simulink model "runGantrySimulink"  (R2025b)
settings: Solver=FixedStepAuto  StartTime=0.0  StopTime=inf  FixedStep=0.05  RelTol=1e-3  EnableMultiTasking=on
libraries: raspberrypiNetworklib x4, raspberrypiBasiclib x4, etargetslib x2
settings Model: ExtModeTrigDuration=2  Creator=ioannisgeorgilas  LastModifiedBy=james
settings SolverCC: PositivePriorityOrder=on
settings OptimizationCC: EnhancedBackFolding=on  PassReuseOutputArgsAs=Individual arguments  ZeroExternalMemoryAtStartup=off  ZeroInternalMemoryAtStartup=off  MaxStackSize=200000  OptimizeBlockOrder=speed  DifferentSizesBufferReuse=on  OptimizationCustomize=off  EfficientTunableParamExpr=on
settings DebuggingCC: ParameterTunabilityLossMsg=error
settings HardwareCC: ProdBitPerPointer=32.0  ProdBitPerSizeT=32.0  ProdBitPerPtrDiffT=32.0  ProdLargestAtomicInteger=Long  ProdLargestAtomicFloat=Double  ProdWordSize=32.0  ProdLongLongMode=on  ProdHWDeviceType=ARM Compatible->ARM Cortex-A (32-bit)
settings RTWCC: SystemTargetFile=ert.tlc  HardwareBoard=Raspberry Pi  TLCOptions="-aInlineSetEventsForThisBaseRateFcn=TLC_FALSE -aSuppressMultiTaskScheduler=TLC_FALSE  -aRateBasedStepFcn=0"  TemplateMakefile=ert_default_tmf  Toolchain=GNU GCC Embedded Linux  BuildConfiguration=Faster Runs  Description=Embedded Coder
settings CodeAppCC: ForceParamTrailComments=on  IgnoreCustomStorageClasses=off  OperatorAnnotations=on  SimulinkDataObjDesc=on  SFDataObjDesc=on  InsertBlockDesc=on
settings ERTTargetCC: ExtModeTransport=2.0  ExtModeStaticAlloc=on  ExtModeMexFile=ext_xcp  ExtModeIntrfLevel=Level2 - Open  InlinedParameterPlacement=Hierarchical  CodeReplacementLibrary=ARM Cortex-A CMSIS  SupportContinuousTime=on  SupportVariableSizeSignals=on

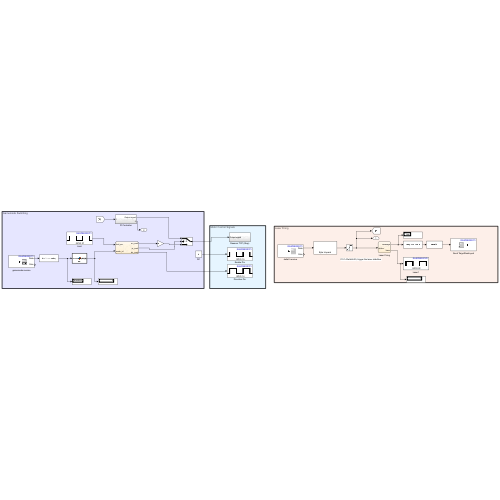
[thumbnail: Simulink's stored preview of the top-level diagram]
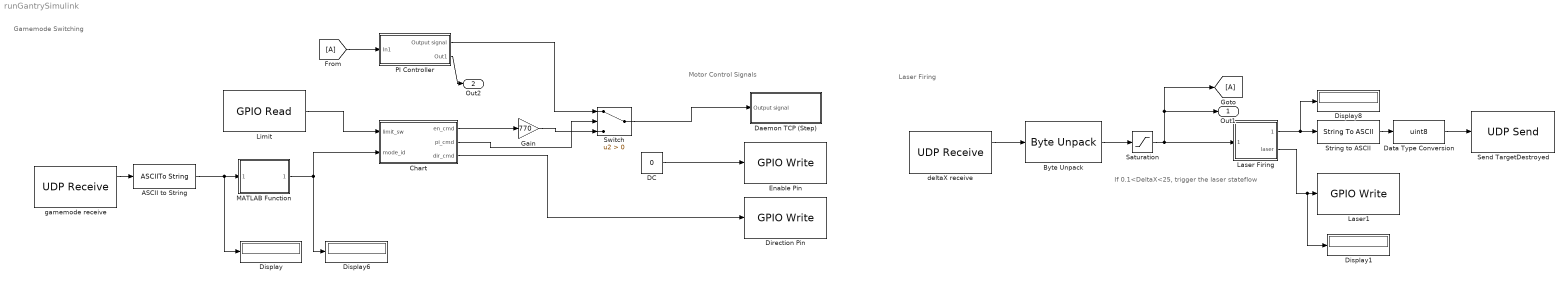
== system runGantrySimulink ==
  note: If 0.1<DeltaX<25, trigger the laser stateflow
  note: Motor Control Signals
  note: Laser Firing
  note: Gamemode Switching
  ASCII to String : ASCIIToString
  Byte Unpack : etargetslib/Byte Unpack  dimensions={[1]}  datatypes={'int32'}  byteAlign=1
      settings: LibrarySourceBlock=embeddedtargetslib/Host Communication/Byte Unpack
  Chart : Stateflow chart  TreatAsAtomicUnit=on
  DC : Constant  Value=0
  Daemon TCP (Step) : Subsystem
  Data Type Conversion : DataTypeConversion  OutDataTypeStr=uint8  SaturateOnIntegerOverflow=off  RndMeth=Floor
  Direction Pin : raspberrypiBasiclib/GPIO Write  BoardProperty=Pi Zero 2 W  gpio=14  blockPlatform=Raspberry Pi  PinNumber=17  board=[]  direction=[]
  Display{,1,6,8} (4 alike) : Display
  Enable Pin : raspberrypiBasiclib/GPIO Write  BoardProperty=Pi Zero 2 W  gpio=15  blockPlatform=Raspberry Pi  PinNumber=17  board=[]  direction=[]
  From : From
  Gain : Gain  Gain=770
  Goto : Goto
  Laser Firing : Stateflow chart  TreatAsAtomicUnit=on
  Laser1 : raspberrypiBasiclib/GPIO Write  BoardProperty=Pi Zero 2 W  gpio=22  blockPlatform=Raspberry Pi  PinNumber=17  board=[]  direction=[]
  Limit : raspberrypiBasiclib/GPIO Read  BoardProperty=Pi Zero 2 W  gpio=27  SampleTime=0.05  blockPlatform=Raspberry Pi  PinNumber=4  board=[]  direction=[]  internalResistor=[]
  MATLAB Function : MATLAB Function  TreatAsAtomicUnit=on
  PI Controller : Subsystem
  Saturation : Saturate  UpperLimit=500  LowerLimit=-500
  Send TargetDestroyed : raspberrypiNetworklib/UDP Send  remoteURL='172.26.236.65'  remotePort=55004  localURL='0.0.0.0'  localPortSource=Automatically determine  localPort=-1  sampletime=-1  blockPlatform=Raspberry Pi  separateLengthPort=0
  String to ASCII : StringToASCII
  Switch : Switch  Criteria=u2 > Threshold  SaturateOnIntegerOverflow=off  InputSameDT=off
  deltaX receive : raspberrypiNetworklib/UDP Receive  localURL='0.0.0.0'  localPort=55010  remoteURL='0.0.0.0'  remotePort=-1  recvBufferSize=8192  signalDatatype=uint8  dims=4  isVarSize=off  showBlockingTime=off  blockingTime=0  sampletime=0.05  blockPlatform=Raspberry Pi
  gamemode receive : raspberrypiNetworklib/UDP Receive  localURL='0.0.0.0'  localPort=50001  remoteURL='0.0.0.0'  remotePort=-1  recvBufferSize=8192  signalDatatype=uint8  dims=14  isVarSize=off  showBlockingTime=off  blockingTime=0  sampletime=0.05  blockPlatform=Raspberry Pi
  Out1 : Outport
  Out2 : Outport  Port=2
  wires:
  Chart/3(dir_cmd) -> Direction Pin/1
  ASCII to String/1 -> MATLAB Function/1(command_string), Display/1
  Limit/1 -> Chart/1(limit_sw)
  DC/1 -> Enable Pin/1
  MATLAB Function/1(mode_id) -> Chart/2(mode_id), Display6/1
  gamemode receive/1 -> ASCII to String/1
  deltaX receive/1 -> Byte Unpack/1
  Byte Unpack/1 -> Saturation/1
  Saturation/1 -> Laser Firing/1(deltax), Goto/1, Out1/1
  Data Type Conversion/1 -> Send TargetDestroyed/1
  Laser Firing/1(message) -> Display8/1, String to ASCII/1
  String to ASCII/1 -> Data Type Conversion/1
  Chart/2(pi_cmd) -> Switch/2
  PI Controller/1(Output signal) -> Switch/1
  PI Controller/2(Out1) -> Out2/1
  Switch/1 -> Daemon TCP (Step)/1(Output signal)
  Chart/1(en_cmd) -> Gain/1
  Gain/1 -> Switch/3
  From/1 -> PI Controller/1(In1)
  Laser Firing/2(laser) -> Display1/1, Laser1/1

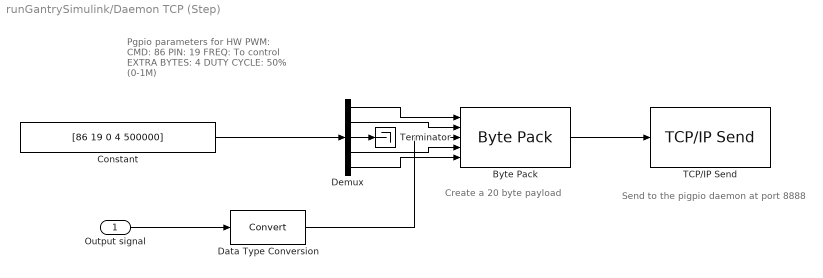
== system runGantrySimulink/Daemon TCP (Step) ==
  note: Pgpio parameters for HW PWM:
      | CMD: 86
      | PIN: 19
      | FREQ: To control
      | EXTRA BYTES: 4
      | DUTY CYCLE: 50% (0-1M)
  note: Create a 20 byte payload
  note: Send to the pigpio daemon at port 8888
  Output signal : Inport
  Byte Pack : etargetslib/Byte Pack  datatypes={'uint32','uint32','uint32','uint32','uint32'}  byteAlign=1
  Constant : Constant  Value=[86 19 0 4 500000]  OutDataTypeStr=Inherit: Inherit via back propagation
  Data Type Conversion : DataTypeConversion  SaturateOnIntegerOverflow=off  RndMeth=Floor
  Demux : Demux  Outputs=5
  TCP/IP Send : raspberrypiNetworklib/TCP//IP Send  Mode_=Client  LocalServerPort_=25000  RemoteAddr_=127.0.0.1  RemoteServerPort_=8888  SimulateUsing=Code generation  ClientPortBindingSelection_=off  ClientPortToBind_=35000  BlockingMode_=off  BlockTimeout_=0.1  BlockPlatform=RASPBERRYPI
  Terminator : Terminator
  wires:
  Byte Pack/1 -> TCP/IP Send/1
  Demux/1 -> Byte Pack/1
  Demux/2 -> Byte Pack/2
  Demux/3 -> Terminator/1
  Demux/4 -> Byte Pack/4
  Demux/5 -> Byte Pack/5
  Data Type Conversion/1 -> Byte Pack/3
  Constant/1 -> Demux/1
  Output signal/1 -> Data Type Conversion/1

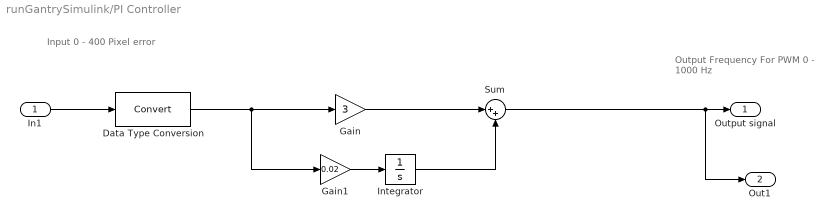
== system runGantrySimulink/PI Controller ==
  note: Output Frequency For PWM
      | 0 - 1000 Hz
  note: Input 0 - 400 Pixel error
  In1 : Inport
  Data Type Conversion : DataTypeConversion  SaturateOnIntegerOverflow=off  RndMeth=Floor
  Gain : Gain  Gain=3
  Gain1 : Gain  Gain=0.02
  Integrator : Integrator
  Sum : Sum  Inputs=|++
  Output signal : Outport
  Out1 : Outport  Port=2
  wires:
  Data Type Conversion/1 -> Gain1/1, Gain/1
  Gain1/1 -> Integrator/1
  Gain/1 -> Sum/1
  Integrator/1 -> Sum/2
  Sum/1 -> Out1/1, Output signal/1
  In1/1 -> Data Type Conversion/1

== stateflow chart runGantrySimulink/Laser Firing ==
  state Idle
    entry: laser = 0;
    entry: message = "Idle";
  state Fire
    entry: laser = 1;
    entry: message = "Firing";
  state Send
    entry: message = "Target Destroyed";
    entry: laser = 0;
  (default) -> Idle
  Idle -> Fire : [deltax > 5 && deltax < 25]
  Send -> Idle : after(5, sec)
  Fire -> Send : [deltax > 25 || deltax < 6]
  data: message output string ="Idle"; laser output =0; deltax input

== matlab function runGantrySimulink/MATLAB Function ==
  data: command_string input; mode_id output
function mode_id = fcn(command_string)
    % Input: command_string (from 'ASCII to String' block)
    % Output: Integer ID for Stateflow
    
    % Convert the Simulink string to a character array
    cmd_chars = char(command_string);
    
    % Safety Check: If empty, do nothing (Idle)
    if isempty(cmd_chars)
        mode_id = 0;
        return;
    end
    
    % Grab just the first letter
    first_letter = cmd_chars(1);
    
    % Check logic
    if first_letter == 'i'      % i = idle
        mode_id = 0;
        
    elseif first_letter == 'c'  % c = calibrate
        mode_id = 1;
        
    elseif first_letter == 's'  % f = selection
        mode_id = 2;
        
    elseif first_letter == 'a'  % a = attack
        mode_id = 3;
        
    elseif first_letter == 'e'  % e = end
        mode_id = 4;
        
    else
        % Default to Idle if unknown
        mode_id = 0; 
    end
end

== stateflow chart runGantrySimulink/Chart ==
  state Active
    state MoveAway
      entry: en_cmd = 1;
      entry: dir_cmd = 1;
      entry: pi_cmd = 0;
    state MoveHome
      entry: en_cmd = 1;
      entry: dir_cmd = 0;
      entry: pi_cmd = 0;
    state idle
      entry: en_cmd = 0;
      entry: dir_cmd = 0;
      entry: pi_cmd = 0;
    state Attack
      entry: en_cmd = 0;
      entry: dir_cmd = 0;
      entry: pi_cmd = 1;
    state idle1
      entry: en_cmd = 0;
      entry: dir_cmd = 0;
      entry: pi_cmd = 0;
    state Finding
      entry: en_cmd = 1;
      entry: dir_cmd = 1;
      entry: pi_cmd = 0;
    state idle2
      entry: en_cmd = 0;
      entry: dir_cmd = 0;
      entry: pi_cmd = 0;
    idle -> MoveAway : [mode_id == 1]
    MoveAway -> MoveHome : after(2, sec)
    (default) -> idle
    Attack -> idle : [mode_id == 0]
    MoveHome -> idle1 : [limit_sw == 0]
    idle2 -> Attack : [mode_id == 3]
    idle1 -> Finding : [mode_id == 2]
    Finding -> idle2 : after(10, sec)
  state Emergency_Stop
    entry: en_cmd = 0;
    entry: dir_cmd = 1;
    entry: pi_cmd = 0;
  (default) -> Active
  Emergency_Stop -> Active : [mode_id == 0]
  Active -> Emergency_Stop : [limit_sw == 0 && mode_id ~= 0 && mode_id ~= 1 && mode_id ~= 2]
  data: limit_sw input; en_cmd output double =1; pi_cmd output; dir_cmd output =1; mode_id input
